simulink model "try_vpasolve"  (R2021a)
settings: Solver=VariableStepAuto  StartTime=0.0  StopTime=10.0  RelTol=1e-3
settings Model: Creator=tejal  LastModifiedBy=tejal

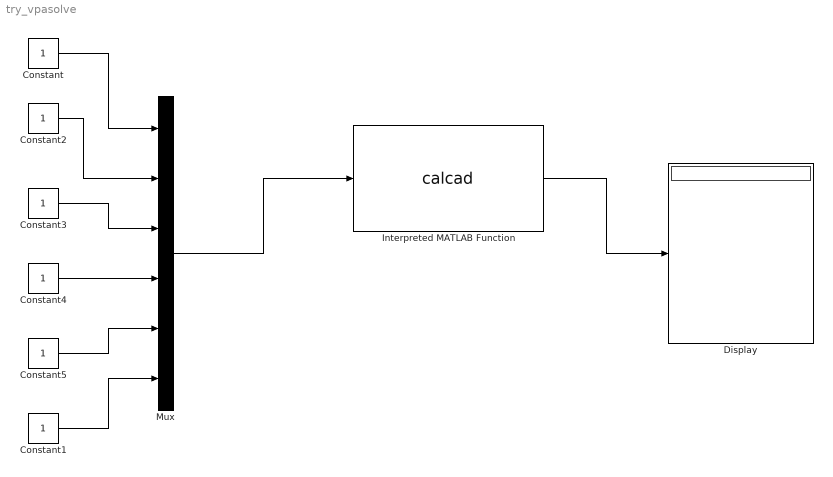
== system try_vpasolve ==
  Constant{,1..5} (6 alike) : Constant
  Display : Display
  Interpreted MATLAB Function : MATLABFcn  MATLABFcn=calcad  OutputDimensions=2
  Mux : Mux  Inputs=6
  wires:
  Constant/1 -> Mux/1
  Constant2/1 -> Mux/2
  Constant3/1 -> Mux/3
  Constant4/1 -> Mux/4
  Constant5/1 -> Mux/5
  Constant1/1 -> Mux/6
  Mux/1 -> Interpreted MATLAB Function/1
  Interpreted MATLAB Function/1 -> Display/1
